simulink model "problem_3"  (R2020b)
settings: Solver=VariableStepAuto  StartTime=0.0  StopTime=10.0  RelTol=1e-3
PreLoadFcn:
  | vars
values from neighbouring files (symbols this model uses):
  g = 32.1800    (= 32.18)    [vars.m]
  Kf = 1    [vars.m]
  m = 50    [vars.m]
  mu = [0 0.4 0.8 0.97 1 0.98 0.96 0.94 0.92 0.9 0.88 0.855 0.83 0.81 0.79 0.77 0.75 0.73 0.72 0.71 0.7]    [vars.m]
  PBmax = 1500    [vars.m]
  Rr = 1.25    [vars.m]
  slip = [0 0.05 0.1 0.15000000000000002 0.2 0.25 0.30000000000000004 0.35000000000000003 0.4 0.45 0.5 0.55 0.6 0.64999999999999991 0.7 0.75 0.8 0.85 0.9 0.95 1]    [vars.m]
  TB = 0.0100    (= 0.01)    [vars.m]
  v0 = 88    [vars.m]
settings Model: Creator=hp  LastModifiedBy=hp

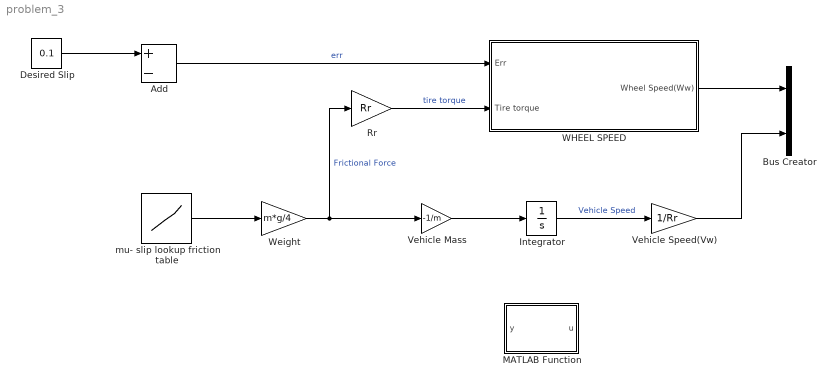
== system problem_3 ==
  Add : Sum  Inputs=+-
  Bus Creator : BusCreator  Inputs=2
  Desired Slip : Constant  Value=0.1
  Integrator : Integrator  InitialCondition=v0  LimitOutput=on  UpperSaturationLimit=1000  LowerSaturationLimit=0
  MATLAB Function : MATLAB Function  TreatAsAtomicUnit=on
  Rr : Gain  Gain=Rr  SaturateOnIntegerOverflow=on  OutDataTypeStr=Inherit: Same as input  ParamDataTypeStr=Inherit: Same as input
  Vehicle Mass : Gain  Gain=-1/m
  Vehicle Speed(Vw) : Gain  Gain=1/Rr
  WHEEL SPEED : Subsystem
  Weight : Gain  Gain=m*g/4  SaturateOnIntegerOverflow=on  OutDataTypeStr=Inherit: Same as input  ParamDataTypeStr=Inherit: Same as input
  mu- slip lookup friction table : Lookup_n-D  NumberOfTableDimensions=1  BreakpointsForDimension1=slip  Table=mu  InternalRulePriority=Speed  RndMeth=Simplest  InputSameDT=on
  wires:
  Desired Slip/1 -> Add/1
  Add/1 -> WHEEL SPEED/1(Err)  "err"
  mu- slip lookup friction table/1 -> Weight/1
  Rr/1 -> WHEEL SPEED/2(Tire torque)  "tire torque"
  Weight/1 -> Vehicle Mass/1, Rr/1  "Frictional Force"
  Vehicle Mass/1 -> Integrator/1
  Integrator/1 -> Vehicle Speed(Vw)/1  "Vehicle Speed"
  WHEEL SPEED/1(Wheel Speed(Ww)) -> Bus Creator/1
  Vehicle Speed(Vw)/1 -> Bus Creator/2

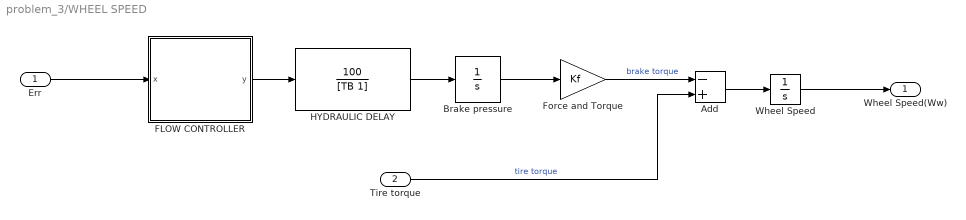
== system problem_3/WHEEL SPEED ==
  Err : Inport
  Tire torque : Inport  Port=2
  Add : Sum  Inputs=-+
  Brake pressure : Integrator  LimitOutput=on  UpperSaturationLimit=PBmax  LowerSaturationLimit=0
  FLOW CONTROLLER : Stateflow chart  TreatAsAtomicUnit=on
  Force and Torque : Gain  Gain=Kf
  HYDRAULIC DELAY : TransferFcn  Numerator=[100]  Denominator=[TB 1]
  Wheel Speed : Integrator  InitialCondition=v0/Rr  LimitOutput=on  UpperSaturationLimit=1000  LowerSaturationLimit=0
  Wheel Speed(Ww) : Outport
  wires:
  Err/1 -> FLOW CONTROLLER/1(x)
  FLOW CONTROLLER/1(y) -> HYDRAULIC DELAY/1
  HYDRAULIC DELAY/1 -> Brake pressure/1
  Brake pressure/1 -> Force and Torque/1
  Force and Torque/1 -> Add/1  "brake torque"
  Tire torque/1 -> Add/2  "tire torque"
  Add/1 -> Wheel Speed/1
  Wheel Speed/1 -> Wheel Speed(Ww)/1

== matlab function problem_3/MATLAB Function ==
  data: u input; y output
function y = fcn(u)

y = 1.0 - u(1)/(u(2) + (u(2)==0)*eps);

== stateflow chart problem_3/WHEEL SPEED/FLOW CONTROLLER ==
  (default) -> (junction 7) : % Control for +1 or -1 for error input
  (junction 7) -> (junction 8) [order 1] : [x>0]
  (junction 7) -> (junction 9) [order 2] : {y=-x;}
  (junction 8) -> (junction 10) : {y=x;}
  (junction 10) -> (junction 9)
  (junction 9) -> (junction 11)
  data: x input; y output
